simulink model "PNT_Unit"  (R2020b)
settings: configuration reference "unit_config" (kept outside this file)
libraries: simulink_extras x1
settings Model: DataDictionary=Hybrid_vehicle_update.sldd  SimulationMode=accelerator  Creator=Georg  LastModifiedBy=jy
settings ConfigSetRef: SourceName=unit_config

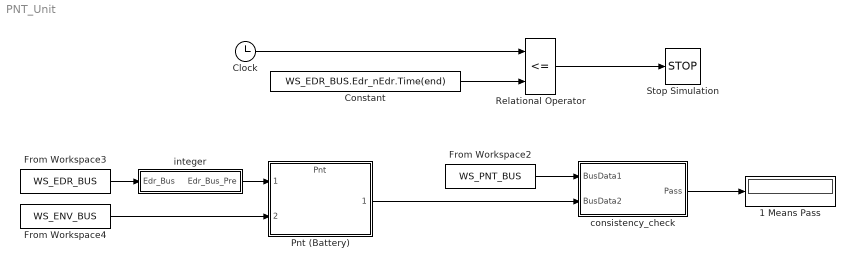
== system PNT_Unit ==
  1 Means Pass : Display
  Clock : Clock
  Constant : Constant  Value=WS_EDR_BUS.Edr_nEdr.Time(end)
  From Workspace2 : FromWorkspace  VariableName=WS_PNT_BUS  OutDataTypeStr=Bus: PNT_BUS  SampleTime=0.002  Interpolate=off  OutputAfterFinalValue=Holding final value
  From Workspace3 : FromWorkspace  VariableName=WS_EDR_BUS  OutDataTypeStr=Bus: EDR_BUS  SampleTime=0.002  Interpolate=off  OutputAfterFinalValue=Holding final value
  From Workspace4 : FromWorkspace  VariableName=WS_ENV_BUS  OutDataTypeStr=Bus: ENV_BUS  SampleTime=0.002  Interpolate=off  OutputAfterFinalValue=Holding final value
  Pnt (Battery) : ModelReference  ModelNameDialog=Pnt  SimulationMode=Normal  ModelReferenceVersion=2.20
      mask Display: image('C:\git\Unit-models-in-Simulink-MIL-tests\updated_structure\img\Battery.jpg'); % Use "Edit Image" on toolstrip to change.
  Relational Operator : RelationalOperator  Operator=<=  OutDataTypeStr=boolean  RndMeth=Simplest
  Stop Simulation : Stop
  consistency_check : Subsystem
  integer : Subsystem
  wires:
  consistency_check/1(Pass) -> 1 Means Pass/1
  Clock/1 -> Relational Operator/1
  Relational Operator/1 -> Stop Simulation/1
  Constant/1 -> Relational Operator/2
  From Workspace2/1 -> consistency_check/1(BusData1)
  From Workspace3/1 -> integer/1(Edr_Bus)
  integer/1(Edr_Bus_Pre) -> Pnt (Battery)/1
  From Workspace4/1 -> Pnt (Battery)/2
  Pnt (Battery)/1 -> consistency_check/2(BusData2)

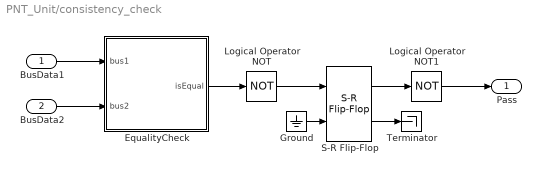
== system PNT_Unit/consistency_check ==
  BusData1 : Inport
  BusData2 : Inport  Port=2
  EqualityCheck : MATLAB Function  TreatAsAtomicUnit=on
  Ground : Ground
  Logical Operator NOT : Logic  Operator=NOT  AllPortsSameDT=off  OutDataTypeStr=boolean
  Logical Operator NOT1 : Logic  Operator=NOT  AllPortsSameDT=off  OutDataTypeStr=boolean
  S-R Flip-Flop : simulink_extras/Flip Flops/S-R Flip-Flop  initial_condition=0
  Terminator : Terminator
  Pass : Outport  VectorParamsAs1DForOutWhenUnconnected=off
  wires:
  BusData1/1 -> EqualityCheck/1(bus1)
  BusData2/1 -> EqualityCheck/2(bus2)
  EqualityCheck/1(isEqual) -> Logical Operator NOT/1
  Logical Operator NOT/1 -> S-R Flip-Flop/1
  Ground/1 -> S-R Flip-Flop/2
  S-R Flip-Flop/2 -> Terminator/1
  S-R Flip-Flop/1 -> Logical Operator NOT1/1
  Logical Operator NOT1/1 -> Pass/1

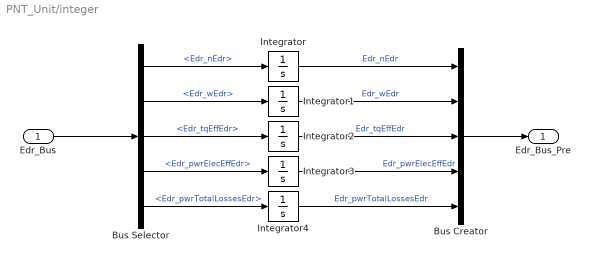
== system PNT_Unit/integer ==
  Edr_Bus : Inport  OutDataTypeStr=Bus: EDR_BUS
  Bus Creator : BusCreator  Inputs=5
  Bus Selector : BusSelector  OutputSignals=Edr_nEdr,Edr_wEdr,Edr_tqEffEdr,Edr_pwrElecEffEdr,Edr_pwrTotalLossesEdr
  Integrator{,1..4} (5 alike) : Integrator
  Edr_Bus_Pre : Outport  OutDataTypeStr=Bus: EDR_BUS
  wires:
  Edr_Bus/1 -> Bus Selector/1
  Integrator3/1 -> Bus Creator/4  "Edr_pwrElecEffEdr"
  Integrator/1 -> Bus Creator/1  "Edr_nEdr"
  Bus Creator/1 -> Edr_Bus_Pre/1
  Integrator1/1 -> Bus Creator/2  "Edr_wEdr"
  Integrator2/1 -> Bus Creator/3  "Edr_tqEffEdr"
  Integrator4/1 -> Bus Creator/5  "Edr_pwrTotalLossesEdr"
  Bus Selector/1 -> Integrator/1  "<Edr_nEdr>"
  Bus Selector/2 -> Integrator1/1  "<Edr_wEdr>"
  Bus Selector/3 -> Integrator2/1  "<Edr_tqEffEdr>"
  Bus Selector/4 -> Integrator3/1  "<Edr_pwrElecEffEdr>"
  Bus Selector/5 -> Integrator4/1  "<Edr_pwrTotalLossesEdr>"

== matlab function PNT_Unit/consistency_check/EqualityCheck ==
  data: bus1 input; isEqual output; bus2 input
function isEqual = fcn(bus1, bus2)
isEqual = isequal(bus1, bus2);
